simulink model "communicationTesting"  (R2024b)
settings: Solver=VariableStepAuto  StartTime=0.0  StopTime=10.0  RelTol=1e-3
undefined symbols (not defined in the file or in its folder): localhost
libraries: simulink x2, modbuslib x2
settings Model: Creator=aidan  LastModifiedBy=aidan

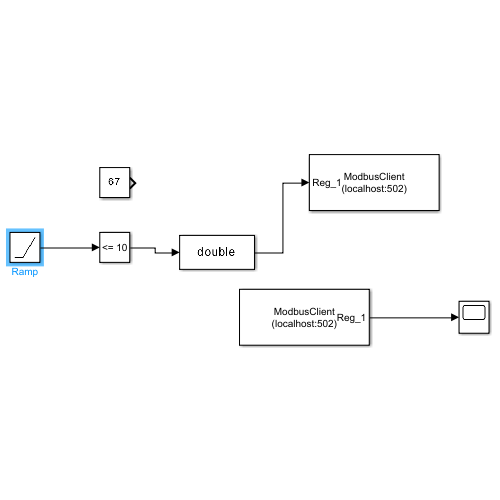
[thumbnail: Simulink's stored preview of the top-level diagram]
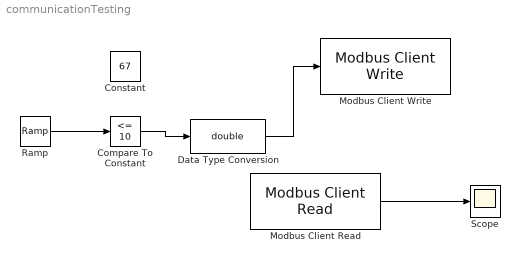
== system communicationTesting ==
  Compare To Constant : simulink/Logic and Bit Operations/Compare To Constant  relop=<=  const=10  OutDataTypeStr=boolean
  Constant : Constant  Value=67
  Data Type Conversion : DataTypeConversion  OutMin=0  OutMax=1  OutDataTypeStr=double  SaturateOnIntegerOverflow=off  RndMeth=Floor
  Modbus Client Read : modbuslib/Modbus Client Read  RetainClient=ModbusClient  ClientList=ModbusClient  ConnectionEndpoint=localhost:502  ServerId=1  RegisterTable={ '1', 'Reg_1', '1', 'Holding Register', 'uint16', '1' }  SampleTime=0.1
  Modbus Client Write : modbuslib/Modbus Client Write  RetainClient=ModbusClient  ClientList=ModbusClient  ConnectionEndpoint=localhost:502  ServerId=1  RegisterTable={ '1', 'Reg_1', '5', 'Holding Register', 'uint16' }  SampleTime=-1
  Ramp : simulink/Sources/Ramp  slope=2  start=0  InitialOutput=0
  Scope : Scope
  wires:
  Modbus Client Read/1 -> Scope/1
  Ramp/1 -> Compare To Constant/1
  Compare To Constant/1 -> Data Type Conversion/1
  Data Type Conversion/1 -> Modbus Client Write/1
